simulink model "first_basic_SMC"  (R2024b)
settings: Solver=VariableStepAuto  StartTime=0.0  StopTime=10  RelTol=1e-3
libraries: slpidlib x1, simulink_extras x1
settings Model: Creator=ayush  LastModifiedBy=ayush

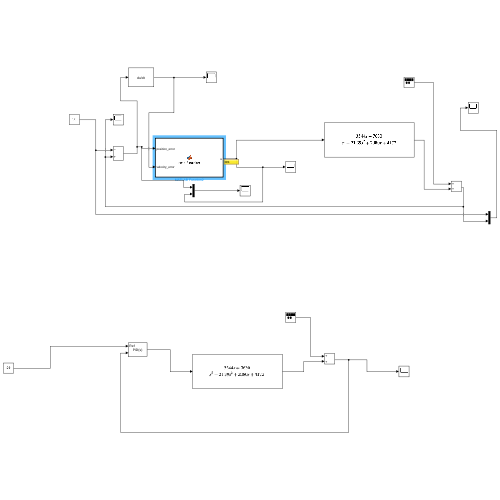
[thumbnail: Simulink's stored preview of the top-level diagram]
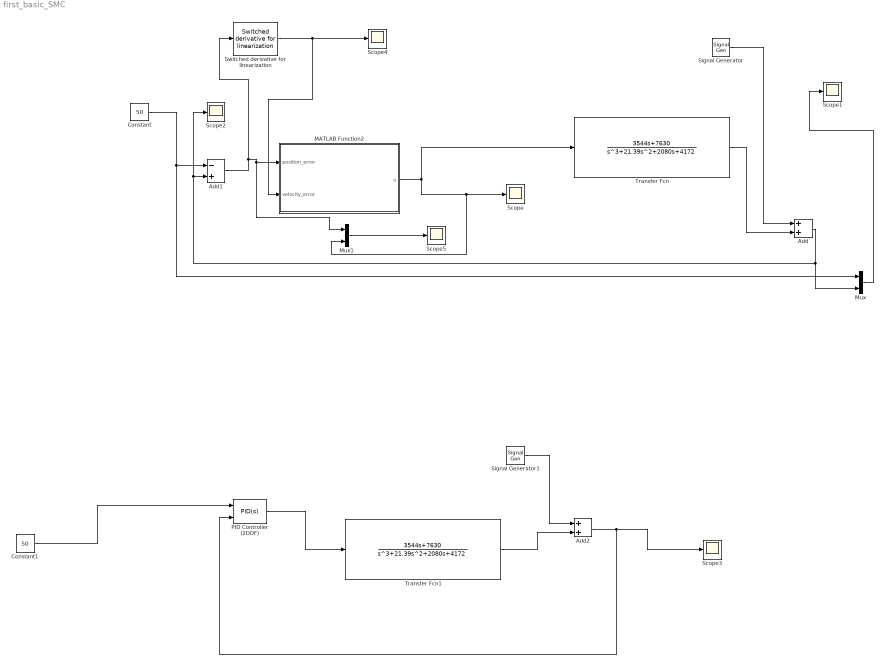
== system first_basic_SMC ==
  Add : Sum
  Add1 : Sum  Inputs=-+
  Add2 : Sum
  Constant : Constant  Value=50
  Constant1 : Constant  Value=50
  MATLAB Function2 : MATLAB Function  TreatAsAtomicUnit=on
  Mux : Mux  Inputs=2
  Mux1 : Mux  Inputs=2
  PID Controller (2DOF) : slpidlib/PID Controller (2DOF)  Controller=PID  Form=Parallel  TimeDomain=Continuous-time  UseExternalTs=off  SampleTime=-1  IntegratorMethod=Forward Euler  FilterMethod=Forward Euler  ControllerParametersSource=internal  P=0  I=5.23289491530193  UseKiTs=off  D=0  UseExternalDerivativeSource=off  N=100  UseFilter=on  b=1  c=1  TunerSelectOption=Transfer Function Based (PID Tuner App)  InitialConditionSource=internal  InitialConditionForIntegrator=0  InitialConditionForFilter=0  DifferentiatorICPrevScaledInput=0  ExternalReset=none  TrackingMode=off  Kt=1  LimitOutput=off  SatLimitsSource=internal  UpperSaturationLimit=inf  LowerSaturationLimit=-inf  LinearizeAsGain=on  AntiWindupMode=none  Kb=1  LimitIntegrator=off  UpperIntegratorSaturationLimit=inf  LowerIntegratorSaturationLimit=-inf  POutMin=[]  POutMax=[]  IOutMin=[]  IOutMax=[]  DOutMin=[]  DOutMax=[]  NOutMin=[]  NOutMax=[]  bOutMin=[]  bOutMax=[]  cOutMin=[]  cOutMax=[]  SumOutMin=[]  SumOutMax=[]  SaturationOutMin=[]  SaturationOutMax=[]  PParamMin=[]  PParamMax=[]  IParamMin=[]  IParamMax=[]  DParamMin=[]  DParamMax=[]  NParamMin=[]  NParamMax=[]  bParamMin=[]  bParamMax=[]  cParamMin=[]  cParamMax=[]  KbParamMin=[]  KbParamMax=[]  KtParamMin=[]  KtParamMax=[]  KbOutMin=[]  KbOutMax=[]  KtOutMin=[]  KtOutMax=[]  IntegratorOutMin=[]  IntegratorOutMax=[]  FilterOutMin=[]  FilterOutMax=[]  SumI1OutMin=[]  SumI1OutMax=[]  SumI2OutMin=[]  SumI2OutMax=[]  SumI3OutMin=[]  SumI3OutMax=[]  SumI4OutMin=[]  SumI4OutMax=[]  SumDOutMin=[]  SumDOutMax=[]  Sum1OutMin=[]  Sum1OutMax=[]  Sum2OutMin=[]  Sum2OutMax=[]  Sum3OutMin=[]  Sum3OutMax=[]  DifferentiatorOutMin=[]  DifferentiatorOutMax=[]  FilterDiffOutCoefMin=[]  FilterDiffOutCoefMax=[]  ReciprocalOutMin=[]  ReciprocalOutMax=[]  SumDenOutMin=[]  SumDenOutMax=[]  SumNumOutMin=[]  SumNumOutMax=[]  DivideOutMin=[]  DivideOutMax=[]  UdiffTsProdOutMin=[]  UdiffTsProdOutMax=[]  NTsProdOutMin=[]  NTsProdOutMax=[]  UintegralTsProdOutMin=[]  UintegralTsProdOutMax=[]  UngainTsProdOutMin=[]  UngainTsProdOutMax=[]  ClampingZeroOutDataTypeStr=Inherit: Inherit via back propagation  ClampingZeroOutMin=[]  ClampingZeroOutMax=[]  FilterDenConstantOutDataTypeStr=Inherit: Inherit via back propagation  FilterDenConstantOutMin=[]  FilterDenConstantOutMax=[]  PCopyOutDataTypeStr=Inherit: Inherit via back propagation  PCopyOutMin=[]  PCopyOutMax=[]  NCopyOutDataTypeStr=Inherit: Inherit via back propagation  NCopyOutMin=[]  NCopyOutMax=[]  IntegratorContinuousStateAttributes=''  IntegratorStateMustResolveToSignalObject=off  IntegratorRTWStateStorageClass=Auto  FilterContinuousStateAttributes=''  FilterStateMustResolveToSignalObject=off  FilterRTWStateStorageClass=Auto  ParallelPVariant=InternalParameters  IdealPVariant=Disabled  IVariant=InternalParameters  DVariant=InternalParameters  bVariant=InternalParameters  cVariant=InternalParameters  IntegratorVariant=Continuous  SatVariant=Disabled  AWVariant=Passthrough  PCopyVariant=Disabled  TRVariant=Disabled  FdbkBlocksVariant=Forward  IdealPFdbkVariant=Disabled  SatFdbkVariant=Disabled  DerivativeFilterVariant=ContFilter  NVariant=InternalParameters  NCopyVariant=Disabled  FilterICVariant=InternalICsFilter  IntegratorICVariant=InternalICs  ExternalResetVariant=Disabled  TRSumVariant=Passthrough  SumFdbkVariant=Disabled  SumVariant=Sum_PID  TsampFilterVariant=InternalTs  TsampNgainVariant=Passthrough  TsampIntegralVariant=Disabled_SignalSpec  ExternalSaturationOutDataTypeStr=Inherit: Same as second input  DerivativeSourceVariant=ErrorSignal  PreIntVariant=InternalPreInt
  Scope{,1..5} (6 alike) : Scope
  Signal Generator : SignalGenerator  WaveForm=random  Amplitude=0  Units=rad/sec
  Signal Generator1 : SignalGenerator  WaveForm=random  Units=rad/sec
  Switched derivative for linearization : simulink_extras/Linearization/Switched derivative for linearization  switchVal=0  derivConst=100
  Transfer Fcn : TransferFcn  Numerator=[3544 7630]  Denominator=[1 21.39 2080 4172]
  Transfer Fcn1 : TransferFcn  Numerator=[3544 7630]  Denominator=[1 21.39 2080 4172]
  wires:
  MATLAB Function2/1(u) -> Transfer Fcn/1, Mux1/2, Scope/1
  Signal Generator/1 -> Add/1
  Constant/1 -> Mux/1, Add1/1
  Add/1 -> Scope2/1, Add1/2, Mux/2
  Add1/1 -> Switched derivative for linearization/1, Mux1/1, MATLAB Function2/1(position_error)
  Transfer Fcn/1 -> Add/2
  Mux/1 -> Scope1/1
  Constant1/1 -> PID Controller (2DOF)/1
  PID Controller (2DOF)/1 -> Transfer Fcn1/1
  Signal Generator1/1 -> Add2/1
  Transfer Fcn1/1 -> Add2/2
  Add2/1 -> PID Controller (2DOF)/2, Scope3/1
  Switched derivative for linearization/1 -> MATLAB Function2/2(velocity_error), Scope4/1
  Mux1/1 -> Scope5/1

== matlab function first_basic_SMC/MATLAB Function2 ==
  data: position_error input; u output; velocity_error input
% function s = fcn(x1, x2, integral_error)
%     epsilon = 0.35;  % Boundary Layer
%     Kp = 2.00;       % Proportional
%     K = 1.5;         % Control Gain
%     lambda = 0.25;   % Damping Factor
%     Ki = 0.8;        % Integral Gain
% 
%     s = Kp * x1 + lambda * x1 * sat(x1 / epsilon) + Ki * integral_error
% end
% 
% function y = sat(x)
%     if abs(x) > 1
%         y = sign(x);
%     else
%         y = x;
%     end
% end


% function s = fcn(x1 , x2)
% s = x2 + 20*(abs(x1))^2*sign(x1);
% end
% 

function u = smc_function(position_error, velocity_error)
    %position_error = position_error/50 +position_error;
    
    alpha = 40;
    beta = 300;
    lambda = 5;
    s = velocity_error + lambda*position_error;
    u = -alpha * sqrt(abs(s))*tanh(s/0.01) + (-beta * tanh(s/0.01)); %super twisting
    

    %for s = -15:1:0
    %    u = -alpha * sqrt(abs(s))*tanh(s/0.01) + (-beta * tanh(s/0.01));
    %end
    %if position_error < 1.5 & position_error > 0
    %    u = +0.3;
    %end
    %if position_error > -1.5 & position_error < 0
    %    u=-0.3;
    %end 
end
